simulink model "ballol"  (Simulink 2.00)
settings: Solver=ode45  StartTime=0.0  StopTime=10.0  RelTol=1e-3  AbsTol=1e-6
undefined symbols (not defined in the file): d, g, J, L, m, R
settings Model: ConsistencyChecking=off

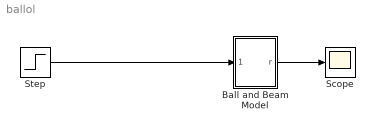
== system ballol ==
  Ball and Beam Model : Subsystem
  Scope : Scope
      settings: TickLabels=on  TimeRange=auto  YMin=-5  YMax=5  SaveToWorkspace=off  SaveName=ScopeData
  Step : Step  Time=0  Before=0  After=1
  wires:
  Step/1 -> Ball and Beam Model/1(theta)
  Ball and Beam Model/1(r) -> Scope/1

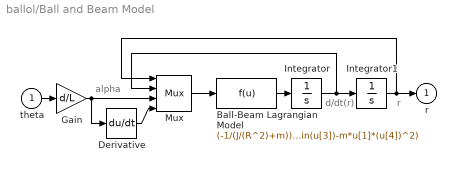
== system ballol/Ball and Beam Model ==
  note: alpha
  note: r
  note: d/dt(r)
  theta : Inport  Port=1  PortWidth=-1  SampleTime=-1
  Ball-Beam Lagrangian Model : Fcn  Expr=(-1/(J/(R^2)+m))*(m*g*sin(u[3])-m*u[1]*(u[4])^2)
  Derivative : Derivative
  Gain : Gain  Gain=d/L
  Integrator : Integrator  ExternalReset=none  InitialConditionSource=internal  InitialCondition=0  LimitOutput=off  UpperSaturationLimit=inf  LowerSaturationLimit=-inf  ShowSaturationPort=off  ShowStatePort=off  AbsoluteTolerance=auto
  Integrator1 : Integrator  ExternalReset=none  InitialConditionSource=internal  InitialCondition=0  LimitOutput=off  UpperSaturationLimit=inf  LowerSaturationLimit=-inf  ShowSaturationPort=off  ShowStatePort=off  AbsoluteTolerance=auto
  Mux : Mux  Inputs=4
  r : Outport  Port=1  InitialOutput=0
  wires:
  Gain/1 -> Mux/3, Derivative/1
  theta/1 -> Gain/1
  Derivative/1 -> Mux/4
  Integrator1/1 -> Mux/1, r/1
  Integrator/1 -> Mux/2, Integrator1/1
  Mux/1 -> Ball-Beam Lagrangian Model/1
  Ball-Beam Lagrangian Model/1 -> Integrator/1
